simulink model "s6"  (R2020b)
settings: Solver=VariableStepAuto  StartTime=0.0  StopTime=10.0  RelTol=1e-3
values from neighbouring files (symbols this model uses):
  A = [0,1,0,0 ... (first row only)    [s6c.m]
  B = [0;1;0;-1.667]    [s6c.m]
  C = [1,0,0,0; 0,0,1,0]    [s6c.m]
  G = place(A',C',PG)'    [s6c.m]
  K = place(A,B,P)    [s6c.m]
settings Model: Creator=huang  LastModifiedBy=huang

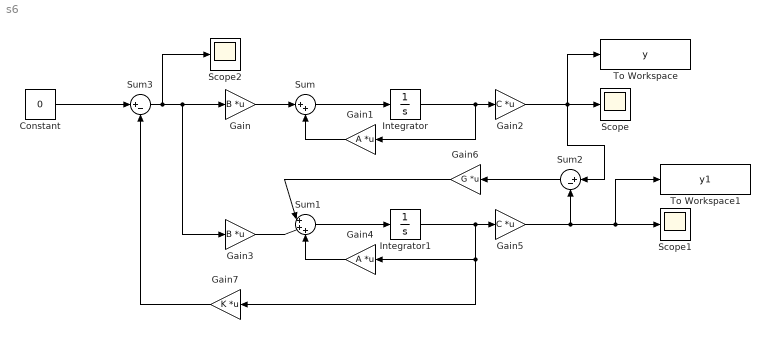
== system s6 ==
  Constant : Constant  Value=0
  Gain : Gain  Gain=B  Multiplication=Matrix(K*u)
  Gain1 : Gain  Gain=A  Multiplication=Matrix(K*u)
  Gain2 : Gain  Gain=C  Multiplication=Matrix(K*u)
  Gain3 : Gain  Gain=B  Multiplication=Matrix(K*u)
  Gain4 : Gain  Gain=A  Multiplication=Matrix(K*u)
  Gain5 : Gain  Gain=C  Multiplication=Matrix(K*u)
  Gain6 : Gain  Gain=G  Multiplication=Matrix(K*u)
  Gain7 : Gain  Gain=K  Multiplication=Matrix(K*u)
  Integrator : Integrator  InitialCondition=[0,0,5,0]'
  Integrator1 : Integrator
  Scope : Scope
  Scope1 : Scope
  Scope2 : Scope
  Sum : Sum  Inputs=|++
  Sum1 : Sum  Inputs=|+++
  Sum2 : Sum  Inputs=|+-
  Sum3 : Sum  Inputs=|+-
  To Workspace : ToWorkspace  VariableName=y  SampleTime=-1
      settings: Save2DSignal=2-D array (concatenate along first dimension)
  To Workspace1 : ToWorkspace  VariableName=y1  SampleTime=-1
      settings: Save2DSignal=2-D array (concatenate along first dimension)
  wires:
  Sum/1 -> Integrator/1
  Gain1/1 -> Sum/2
  Gain/1 -> Sum/1
  Integrator/1 -> Gain1/1, Gain2/1
  Gain2/1 -> Sum2/1, To Workspace/1, Scope/1
  Integrator1/1 -> Gain5/1, Gain7/1, Gain4/1
  Sum1/1 -> Integrator1/1
  Gain5/1 -> To Workspace1/1, Scope1/1, Sum2/2
  Sum2/1 -> Gain6/1
  Gain3/1 -> Sum1/2
  Gain4/1 -> Sum1/3
  Gain6/1 -> Sum1/1
  Sum3/1 -> Scope2/1, Gain3/1, Gain/1
  Gain7/1 -> Sum3/2
  Constant/1 -> Sum3/1
